simulink model "model_inhibth_conditions_safety_module_Test"  (R2024a)
settings: Solver=FixedStepDiscrete  StartTime=0.0  StopTime=10.0  RelTol=1e-3
settings Model: Creator=Gabriel  LastModifiedBy=Gabriel

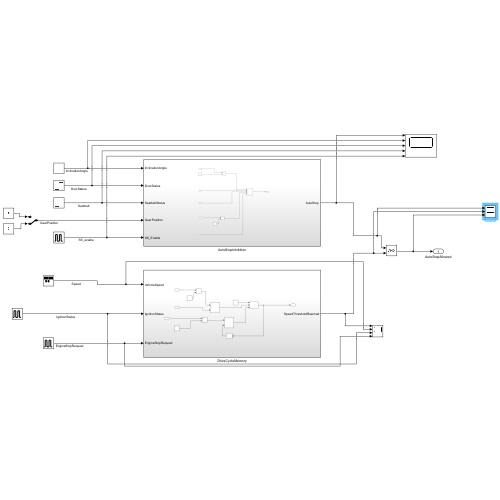
[thumbnail: Simulink's stored preview of the top-level diagram]
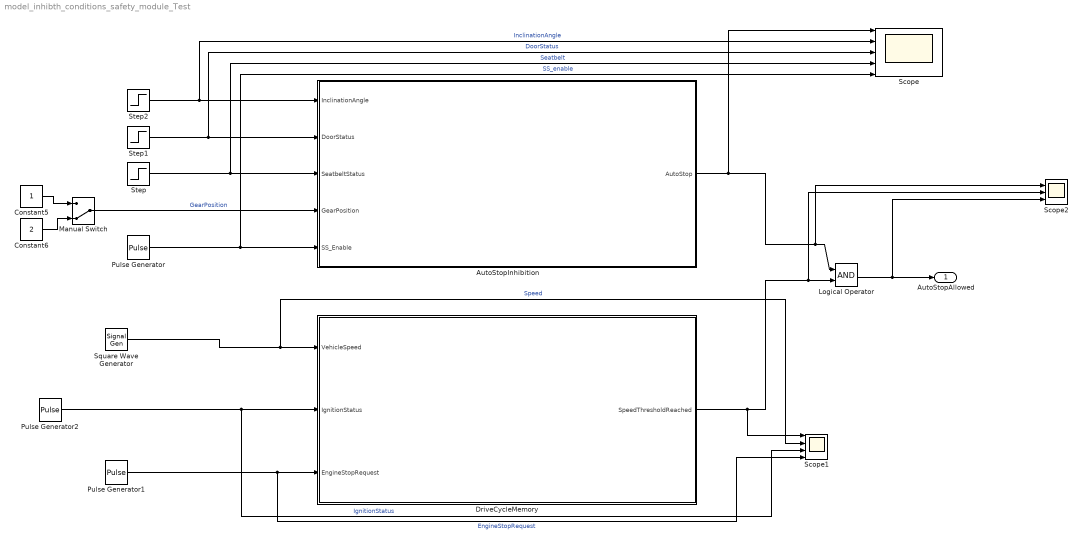
== system model_inhibth_conditions_safety_module_Test ==
  AutoStopInhibition : Subsystem
  Constant5 : Constant
  Constant6 : Constant  Value=2
  DriveCycleMemory : Subsystem
  Logical Operator : Logic  AllPortsSameDT=off  OutDataTypeStr=boolean
  Manual Switch : ManualSwitch  CurrentSetting=0
  Pulse Generator : DiscretePulseGenerator  PulseType=Time based  PulseWidth=70
  Pulse Generator1 : DiscretePulseGenerator  PulseType=Time based  PulseWidth=10
  Pulse Generator2 : DiscretePulseGenerator  PulseType=Time based  PulseWidth=50
  Scope : Scope  NumInputPorts=5
  Scope1 : Scope  NumInputPorts=4
  Scope2 : Scope  NumInputPorts=3
  Square Wave Generator : SignalGenerator  WaveForm=square  Amplitude=10  Units=rad/sec
  Step : Step  Time=4  SampleTime=0
  Step1 : Step  Time=2  SampleTime=0
  Step2 : Step  Time=8  SampleTime=0
  AutoStopAllowed : Outport
  wires:
  Logical Operator/1 -> Scope2/3, AutoStopAllowed/1
  AutoStopInhibition/1("AutoStop ") -> Scope/1, Scope2/1, Logical Operator/1
  DriveCycleMemory/1(SpeedThresholdReached) -> Scope1/1, Scope2/2, Logical Operator/2
  Step2/1 -> Scope/2, AutoStopInhibition/1("InclinationAngle ")  "InclinationAngle"
  Step1/1 -> Scope/3, AutoStopInhibition/2("DoorStatus ")  "DoorStatus"
  Step/1 -> Scope/4, AutoStopInhibition/3("SeatbeltStatus ")  "Seatbelt"
  Pulse Generator/1 -> Scope/5, AutoStopInhibition/5(SS_Enable)  "SS_enable"
  Constant6/1 -> Manual Switch/2
  Constant5/1 -> Manual Switch/1
  Manual Switch/1 -> AutoStopInhibition/4(GearPosition)  "GearPosition"
  Pulse Generator2/1 -> Scope1/3, DriveCycleMemory/2("IgnitionStatus ")  "IgnitionStatus"
  Pulse Generator1/1 -> Scope1/4, DriveCycleMemory/3(EngineStopRequest)  "EngineStopRequest"
  Square Wave Generator/1 -> Scope1/2, DriveCycleMemory/1("VehicleSpeed ")  "Speed"

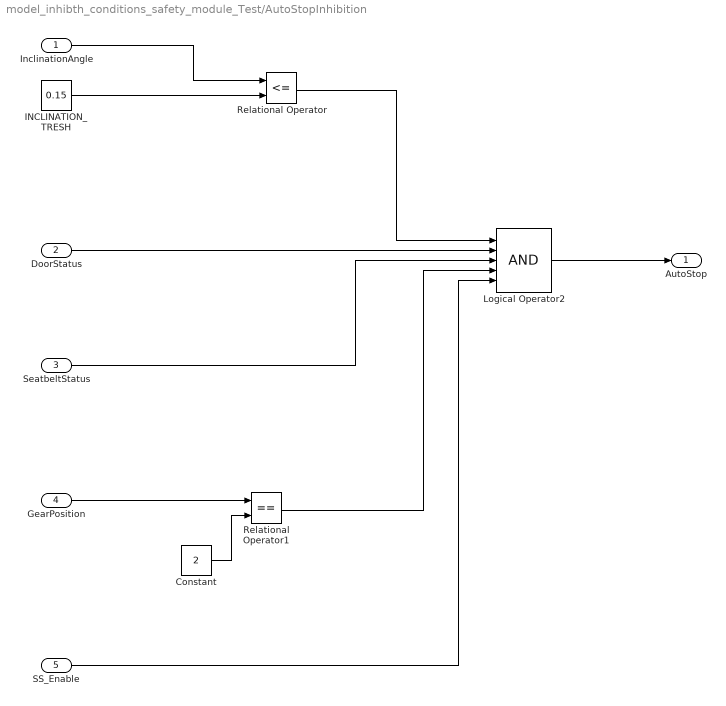
== system model_inhibth_conditions_safety_module_Test/AutoStopInhibition ==
  "InclinationAngle " : Inport
  "DoorStatus " : Inport  Port=2
  "SeatbeltStatus " : Inport  Port=3
  GearPosition : Inport  Port=4
  SS_Enable : Inport  Port=5
  Constant : Constant  Value=2
  INCLINATION_TRESH : Constant  Value=0.15
  Logical Operator2 : Logic  Inputs=5  AllPortsSameDT=off  OutDataTypeStr=boolean
  Relational Operator : RelationalOperator  Operator=<=  OutDataTypeStr=boolean  RndMeth=Simplest  InputSameDT=off
  Relational Operator1 : RelationalOperator  Operator===  OutDataTypeStr=boolean  RndMeth=Simplest  InputSameDT=off
  "AutoStop " : Outport
  wires:
  "DoorStatus "/1 -> Logical Operator2/2
  Logical Operator2/1 -> "AutoStop "/1
  Relational Operator/1 -> Logical Operator2/1
  "SeatbeltStatus "/1 -> Logical Operator2/3
  GearPosition/1 -> Relational Operator1/1
  Relational Operator1/1 -> Logical Operator2/4
  INCLINATION_TRESH/1 -> Relational Operator/2
  "InclinationAngle "/1 -> Relational Operator/1
  Constant/1 -> Relational Operator1/2
  SS_Enable/1 -> Logical Operator2/5

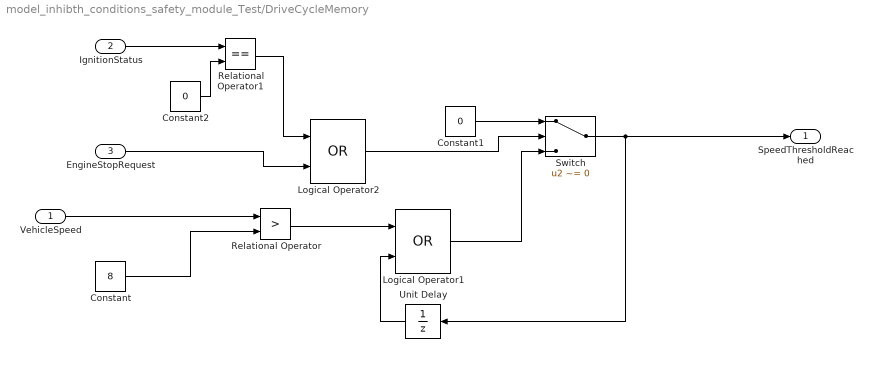
== system model_inhibth_conditions_safety_module_Test/DriveCycleMemory ==
  "VehicleSpeed " : Inport
  "IgnitionStatus " : Inport  Port=2
  EngineStopRequest : Inport  Port=3
  Constant : Constant  Value=8
  Constant1 : Constant  Value=0
  Constant2 : Constant  Value=0
  Logical Operator1 : Logic  Operator=OR  AllPortsSameDT=off  OutDataTypeStr=boolean
  Logical Operator2 : Logic  Operator=OR  AllPortsSameDT=off  OutDataTypeStr=boolean
  Relational Operator : RelationalOperator  Operator=>  OutDataTypeStr=boolean  RndMeth=Simplest  InputSameDT=off
  Relational Operator1 : RelationalOperator  Operator===  OutDataTypeStr=boolean  RndMeth=Simplest  InputSameDT=off
  Switch : Switch  Criteria=u2 ~= 0  SaturateOnIntegerOverflow=off  InputSameDT=off
  Unit Delay : UnitDelay  SampleTime=0.01  HasFrameUpgradeWarning=on
  SpeedThresholdReached : Outport
  wires:
  "VehicleSpeed "/1 -> Relational Operator/1
  Constant/1 -> Relational Operator/2
  Relational Operator/1 -> Logical Operator1/1
  Unit Delay/1 -> Logical Operator1/2
  Constant1/1 -> Switch/1
  Logical Operator1/1 -> Switch/3
  Switch/1 -> Unit Delay/1, SpeedThresholdReached/1
  EngineStopRequest/1 -> Logical Operator2/2
  Logical Operator2/1 -> Switch/2
  "IgnitionStatus "/1 -> Relational Operator1/1
  Constant2/1 -> Relational Operator1/2
  Relational Operator1/1 -> Logical Operator2/1
